simulink library "carnot"  (R2018b)
settings: Solver=VariableStepAuto  StartTime=0.0  StopTime=10.0  RelTol=1e-3
undefined symbols (not defined in the file or in its folder): A, A_earth, acol, Acol, ActPower1, ActPower2, ActPower3, Ad, Ad0, Ar, Au, Au0, Azimuth_Angle, B, Bd, Bd0, Br, Bu, Bu0, C, c1, c2, c3, c33, c4, c5, c6, CarnotCallbacks_Density, CarnotCallbacks_Enthalpy, CarnotCallbacks_Enthalpy2Temperature, CarnotCallbacks_Entropy, CarnotCallbacks_Evaporation_Enthalpy, CarnotCallbacks_GlobalMessageLevel, CarnotCallbacks_Grashof, CarnotCallbacks_Heat_Capacity, CarnotCallbacks_Kinematic_Viscosity, CarnotCallbacks_PMV_PPD, CarnotCallbacks_Prandtl, CarnotCallbacks_Saturation_Property, CarnotCallbacks_Saturation_Temperature, CarnotCallbacks_Saturation_Value_Water, CarnotCallbacks_Specific_Volume, CarnotCallbacks_Thermal_Conductivity, CarnotCallbacks_Vapour_Content, CarnotCallbacks_Vapour_Pressure, Cd, Cdl, Cr, Cu, Davies, Dd, DE_TRY2010_04_averageYear, delta_grd, density, DiameterLastPiece, dl, DPConstant, DPLinear, DPQuadratic, Dr ... (+59)
libraries: $bdroot x429, simulink x36, simulink_extras x12
(part 12 of 22)

== system carnot/Toolbox/Average ==
  input : Inport
  time : Inport  Port=2
  enable : Inport  Port=3
  Demux1 : Demux  Outputs=[-1 1 1]
  Mux : Mux  Inputs=3
  S-Function3 : S-Function  FunctionName=average  Parameters=delta_t offset_flag enable_flag  SFunctionDeploymentMode=off  EnableBusSupport=off  SFcnStateName=D_LAST_OUTPUT
      settings: SFcnIsStateOwnerBlock=on
  average : Outport
  output time : Outport  Port=2
  pulse : Outport  Port=3
  wires:
  Mux/1 -> S-Function3/1
  enable/1 -> Mux/3
  input/1 -> Mux/1
  S-Function3/1 -> Demux1/1
  Demux1/2 -> output time/1
  time/1 -> Mux/2
  Demux1/3 -> pulse/1
  Demux1/1 -> average/1

== system carnot/Toolbox/Economy_Ecology ==
  note: mass of fuel in kg
  note: thermal energy in J
  note: electric energy in J
  note: fuel costs
  note: mass of produced H2O
  note: mass of produced CO2
  note: mass of produced O2
  note: mass of produced SO2
  note: mass of produced N2
  note: mass of produced NOx
  note: mass of produced CO
  note: mass of produced CxHy
  eco : Inport
  Count_Working_Time : $bdroot/Toolbox/Count_Working_Time
  Demux1 : Demux  Outputs=12
  Display : Display
  Integrator : Integrator
  Mux : Mux  Inputs=12
  Mux1 : Mux  Inputs=2
  Selector : Selector  InputPortWidth=16  IndexOptions=Index vector (dialog)  Indices=[3 5:15]  OutputSizes=1
  Selector1 : Selector  InputPortWidth=12  IndexOptions=Index vector (dialog)  Indices=[1]  OutputSizes=1
  Terminator : Terminator
  Terminator1 : Terminator
  Terminator2 : Terminator
  To Workspace : ToWorkspace  VariableName=input_annual_costs  SampleTime=-1
      settings: MaxDataPoints=1
  wires:
  Count_Working_Time/3 -> Terminator2/1
  Count_Working_Time/2 -> Terminator1/1
  Count_Working_Time/1 -> Terminator/1
  Count_Working_Time/4 -> Mux1/2  "Run time"
  Demux1/4 -> Mux1/1, Mux/4  "costs"
  Demux1/1 -> Mux/1  "m_fuel"
  Selector1/1 -> Count_Working_Time/1
  Selector/1 -> Selector1/1, Integrator/1
  Mux1/1 -> To Workspace/1
  Mux/1 -> Display/1
  Demux1/3 -> Mux/3  "E_electric"
  Demux1/2 -> Mux/2  "Qtherm"
  Demux1/10 -> Mux/10  "NOx"
  Demux1/11 -> Mux/11  "CO"
  Demux1/12 -> Mux/12  "CxHy"
  Demux1/9 -> Mux/9  "N2"
  Demux1/6 -> Mux/6  "CO2"
  Integrator/1 -> Demux1/1
  eco/1 -> Selector/1
  Demux1/7 -> Mux/7  "O2"
  Demux1/5 -> Mux/5  "H20"
  Demux1/8 -> Mux/8  "SO2"

== system carnot/Toolbox/GlobalMessageLevel ==

== system carnot/Toolbox/ModelDoc ==

== system carnot/Toolbox/RealDate ==
  S-Function3 : S-Function  FunctionName=systemdate  Parameters=form  SFunctionDeploymentMode=off  EnableBusSupport=off
  date : Outport
  wires:
  S-Function3/1 -> date/1

== system carnot/Toolbox/RealTime ==
  S-Function3 : S-Function  FunctionName=systemtime  SFunctionDeploymentMode=off  EnableBusSupport=off
  time : Outport
  wires:
  S-Function3/1 -> time/1

== system carnot/Toolbox/RealTimePulse ==
  In : Inport
  S-Function : S-Function  FunctionName=monoflop_realtime  Parameters=time typ  SFunctionDeploymentMode=off  EnableBusSupport=off
  Out : Outport
  wires:
  In/1 -> S-Function/1
  S-Function/1 -> Out/1

== system carnot/Toolbox/SystemPulse ==
  enable pulse : Inport
  Mux : Mux  Inputs=2
  S-Function3 : S-Function  FunctionName=systempulse  Parameters=datecheck enable_flag  SFunctionDeploymentMode=off  EnableBusSupport=off
  position6 : Constant  Value=[date period pulsewidth]
  pulse : Outport
  wires:
  Mux/1 -> S-Function3/1
  enable pulse/1 -> Mux/2
  S-Function3/1 -> pulse/1
  position6/1 -> Mux/1

== system carnot/Toolbox/THB2THV ==
  THB : Inport  OutDataTypeStr=Bus: THB
  Bus Selector : BusSelector  OutputSignals=ID,Temperature,MassFlow,Pressure,FluidType,FluidMix,DiameterLastPiece,DPConstant,DPLinear,DPQuadratic,HydraulicInductance,GeodeticHeight,FluidMix2,FluidMix3
  Ground : Ground
  Mux : Mux  Inputs=[1 1 1 1 1 1 1 1 1 1 1 1 1 1 6]
  THV : Outport
  wires:
  Bus Selector/14 -> Mux/14  "<FluidMix3>"
  Bus Selector/13 -> Mux/13  "<FluidMix2>"
  THB/1 -> Bus Selector/1
  Mux/1 -> THV/1
  Bus Selector/1 -> Mux/1  "<ID>"
  Bus Selector/2 -> Mux/2  "<Temperature>"
  Bus Selector/3 -> Mux/3  "<MassFlow>"
  Bus Selector/4 -> Mux/4  "<Pressure>"
  Bus Selector/5 -> Mux/5  "<FluidType>"
  Bus Selector/6 -> Mux/6  "<FluidMix>"
  Bus Selector/7 -> Mux/7  "<DiameterLastPiece>"
  Bus Selector/8 -> Mux/8  "<DPConstant>"
  Bus Selector/9 -> Mux/9  "<DPLinear>"
  Bus Selector/10 -> Mux/10  "<DPQuadratic>"
  Bus Selector/11 -> Mux/11  "<HydraulicInductance>"
  Bus Selector/12 -> Mux/12  "<GeodeticHeight>"
  Ground/1 -> Mux/15

== system carnot/Toolbox/THBMemory ==
  THB_in : Inport  OutDataTypeStr=Bus: THB
  Bus Creator : BusCreator  Inputs=12
  Bus Selector6 : BusSelector  OutputSignals=ID,Temperature,MassFlow,Pressure,FluidType,FluidMix,DiameterLastPiece,DPConstant,DPLinear,DPQuadratic,HydraulicInductance,GeodeticHeight
  Memory_DPConstant : Memory  InitialCondition=c
  Memory_DPLinear : Memory  InitialCondition=l
  Memory_DPQuadratic : Memory  InitialCondition=q
  Memory_DiameterLastPiece : Memory  InitialCondition=d
  Memory_FluidMix : Memory  InitialCondition=FluidMix
  Memory_FluidType : Memory  InitialCondition=FluidType
  Memory_GeodeticHeight : Memory  InitialCondition=H
  Memory_HydraulicInductance : Memory  InitialCondition=LH
  Memory_ID : Memory  InitialCondition=ID
  Memory_MassFlow : Memory  InitialCondition=mdot
  Memory_Pressure : Memory  InitialCondition=p
  Memory_Temperature : Memory  InitialCondition=T
  THB_out : Outport
  wires:
  Bus Selector6/12 -> Memory_GeodeticHeight/1  "<GeodeticHeight>"
  Memory_GeodeticHeight/1 -> Bus Creator/12  "GeodeticHeight"
  Bus Selector6/1 -> Memory_ID/1  "<ID>"
  Memory_ID/1 -> Bus Creator/1  "ID"
  Bus Selector6/2 -> Memory_Temperature/1  "<Temperature>"
  Memory_Temperature/1 -> Bus Creator/2  "Temperature"
  Bus Selector6/3 -> Memory_MassFlow/1  "<MassFlow>"
  Memory_MassFlow/1 -> Bus Creator/3  "MassFlow"
  Bus Selector6/4 -> Memory_Pressure/1  "<Pressure>"
  Memory_Pressure/1 -> Bus Creator/4  "Pressure"
  Bus Selector6/5 -> Memory_FluidType/1  "<FluidType>"
  Memory_FluidType/1 -> Bus Creator/5  "FluidType"
  Bus Selector6/6 -> Memory_FluidMix/1  "<FluidMix>"
  Memory_FluidMix/1 -> Bus Creator/6  "FluidMix"
  Bus Selector6/7 -> Memory_DiameterLastPiece/1  "<DiameterLastPiece>"
  Memory_DiameterLastPiece/1 -> Bus Creator/7  "DiameterLastPiece"
  Bus Selector6/8 -> Memory_DPConstant/1  "<DPConstant>"
  Memory_DPConstant/1 -> Bus Creator/8  "DPConstant"
  Bus Selector6/9 -> Memory_DPLinear/1  "<DPLinear>"
  Memory_DPLinear/1 -> Bus Creator/9  "DPLinear"
  Bus Selector6/10 -> Memory_DPQuadratic/1  "<DPQuadratic>"
  Memory_DPQuadratic/1 -> Bus Creator/10  "DPQuadratic"
  Bus Selector6/11 -> Memory_HydraulicInductance/1  "<HydraulicInductance>"
  Memory_HydraulicInductance/1 -> Bus Creator/11  "HydraulicInductance"
  Bus Creator/1 -> THB_out/1
  THB_in/1 -> Bus Selector6/1

== system carnot/Toolbox/THV2THB ==
  THV : Inport
  Bus Creator : BusCreator  Inputs=14  OutDataTypeStr=Bus: THB
  Demux : Demux  Outputs=[1 1 1 1 1 1 1 1 1 1 1 1 1 1 6]
  Terminator : Terminator
  THB : Outport
  wires:
  [FluidMix3] -> Bus Creator/8  "FluidMix3"
  [FluidMix2] -> Bus Creator/7  "FluidMix2"
  Demux/14 -> [FluidMix3]  "FluidMix3"
  Demux/13 -> [FluidMix2]  "FluidMix2"
  Demux/15 -> Terminator/1
  Demux/12 -> Bus Creator/14  "GeodeticHeight"
  Demux/10 -> Bus Creator/12  "DPQuadratic"
  Demux/9 -> Bus Creator/11  "DPLinear"
  Demux/8 -> Bus Creator/10  "DPConstant"
  Demux/7 -> Bus Creator/9  "DiameterLastPiece"
  Demux/6 -> Bus Creator/6  "FluidMix"
  Demux/5 -> Bus Creator/5  "FluidType"
  Bus Creator/1 -> THB/1
  Demux/4 -> Bus Creator/4  "Pressure"
  Demux/3 -> Bus Creator/3  "MassFlow"
  Demux/1 -> Bus Creator/1  "ID"
  Demux/2 -> Bus Creator/2  "Temperature"
  THV/1 -> Demux/1
  Demux/11 -> Bus Creator/13  "HydraulicInductance"

== system carnot/Toolbox/UnitConv ==
  In : Inport
  S-Function : S-Function  FunctionName=unitconv_s  Parameters=input_unit output_unit  SFunctionDeploymentMode=off  EnableBusSupport=off
  Out : Outport
  wires:
  In/1 -> S-Function/1
  S-Function/1 -> Out/1

== system carnot/Toolbox/UnitConv_Temperature ==
  Tinit : Inport
  S-Function : S-Function  FunctionName=unitconv_temperature_s  Parameters=ini_unit, fin_unit  SFunctionDeploymentMode=off  EnableBusSupport=off
  Tfinal : Outport
  wires:
  S-Function/1 -> Tfinal/1
  Tinit/1 -> S-Function/1

== system carnot/Toolbox/WDB2Weather ==
  WDB : Inport
  Bus Selector1 : BusSelector  OutputSignals=TimeValueComment,Zenith_Angle,Azimuth_Angle,Solar_Radiation_beam_normal,Solar_Radiation_diffuse_horizontal,Temperature_Ambient,Temperature_Sky_Radiation,Relative_Humidity,Precipitation,Cloud_Index,Station_Pressure,Wind_Speed,Wind_Direction,Incidence_Angle_sun,Incidence_Angle_longitudinal,Incidence_Angle_transversal,Solar_Radiation_direct_surface,Solar_Radiation_diffuse_surface
  Mux : Mux  Inputs=18
  weather : Outport
  wires:
  Bus Selector1/1 -> Mux/1  "<TimeValueComment>"
  Bus Selector1/2 -> Mux/2  "<Zenith_Angle>"
  Bus Selector1/3 -> Mux/3  "<Azimuth_Angle>"
  Bus Selector1/4 -> Mux/4  "<Solar_Radiation_beam_normal>"
  Bus Selector1/5 -> Mux/5  "<Solar_Radiation_diffuse_horizontal>"
  Bus Selector1/6 -> Mux/6  "<Temperature_Ambient>"
  Bus Selector1/7 -> Mux/7  "<Temperature_Sky_Radiation>"
  Bus Selector1/8 -> Mux/8  "<Relative_Humidity>"
  Bus Selector1/9 -> Mux/9  "<Precipitation>"
  Bus Selector1/10 -> Mux/10  "<Cloud_Index>"
  Bus Selector1/11 -> Mux/11  "<Station_Pressure>"
  Bus Selector1/12 -> Mux/12  "<Wind_Speed>"
  Bus Selector1/13 -> Mux/13  "<Wind_Direction>"
  Bus Selector1/14 -> Mux/14  "<Incidence_Angle_sun>"
  Bus Selector1/15 -> Mux/15  "<Incidence_Angle_longitudinal>"
  Bus Selector1/16 -> Mux/16  "<Incidence_Angle_transversal>"
  Bus Selector1/17 -> Mux/17  "<Solar_Radiation_direct_surface>"
  Bus Selector1/18 -> Mux/18  "<Solar_Radiation_diffuse_surface>"
  WDB/1 -> Bus Selector1/1
  Mux/1 -> weather/1

== system carnot/Toolbox/Wait ==
  S-Function3 : S-Function  FunctionName=wait  Parameters=date(1) date(2) date(3) date(4) date(5) wtime  SFunctionDeploymentMode=off  EnableBusSupport=off

== system carnot/Toolbox/Weather2WDB ==
  weather : Inport
  Demux : Demux  Outputs=18
  WDB_Creator : $bdroot/Basic/Weather_and_Sun/WDB_Creator
  WDB : Outport
  wires:
  weather/1 -> Demux/1
  WDB_Creator/1 -> WDB/1
  Demux/1 -> WDB_Creator/1  "time_value"
  Demux/2 -> WDB_Creator/2  "zenith"
  Demux/3 -> WDB_Creator/3  "azimuth"
  Demux/4 -> WDB_Creator/4  "I_beam_normal"
  Demux/5 -> WDB_Creator/5  "I_diffuse_horizontal"
  Demux/6 -> WDB_Creator/6  "Tamb"
  Demux/7 -> WDB_Creator/7  "Tsky"
  Demux/8 -> WDB_Creator/8  "relative_humidity"
  Demux/9 -> WDB_Creator/9  "precipitation"
  Demux/10 -> WDB_Creator/10  "cloud_index"
  Demux/11 -> WDB_Creator/11  "pressure"
  Demux/12 -> WDB_Creator/12  "wind_speed"
  Demux/13 -> WDB_Creator/13  "wind_direction"
  Demux/14 -> WDB_Creator/14  "incidence_angle"
  Demux/15 -> WDB_Creator/15  "longitudinal_angle"
  Demux/16 -> WDB_Creator/16  "transversal_angle"
  Demux/17 -> WDB_Creator/17  "I_direct_surface"
  Demux/18 -> WDB_Creator/18  "I_diffuse_surface"

== system carnot/Toolbox/write_txt_file ==
  In : Inport
  enable : Inport  Port=2
  Mux1 : Mux  Inputs=2
  S-Function : S-Function  FunctionName=write_txt_file  Parameters=clear filename  SFunctionDeploymentMode=off  EnableBusSupport=off
  Terminator : Terminator
  wires:
  enable/1 -> Mux1/2
  In/1 -> Mux1/1
  Mux1/1 -> S-Function/1
  S-Function/1 -> Terminator/1

== system carnot/Weather/Add_Solar_Position ==
  WDB_in : Inport
  Bus Assignment : BusAssignment  AssignedSignals=Zenith_Angle,Azimuth_Angle
  Demux : Demux  Outputs=2
  Solar_Position : $bdroot/Basic/Weather_and_Sun/Solar_Position  lati=lati  longi=longi  timezone=timezone
  WDB : Outport
  wires:
  Bus Assignment/1 -> WDB/1
  Demux/2 -> Bus Assignment/3
  Demux/1 -> Bus Assignment/2
  WDB_in/1 -> Bus Assignment/1
  Solar_Position/1 -> Demux/1  "zenith, azimuth"

== system carnot/Weather/DWD_TRY_Radiation_Filter ==
  WDB : Inport
  Bus Assignment : BusAssignment  AssignedSignals=Solar_Radiation_beam_normal,Solar_Radiation_diffuse_horizontal,Solar_Radiation_direct_surface,Solar_Radiation_diffuse_surface
  Bus Selector1 : BusSelector  OutputSignals=Incidence_Angle_sun
  Bus Selector2 : BusSelector  OutputSignals=Solar_Radiation_beam_normal,Solar_Radiation_diffuse_horizontal,Solar_Radiation_direct_surface,Solar_Radiation_diffuse_surface
  Degrees to Radians : simulink_extras/Transformations/Degrees to Radians
  Demux : Demux  Outputs=3
  Gain : Gain  Gain=f
  MinMax : MinMax  Inputs=2
  Mux : Mux  Inputs=3
  Product : Product
  Saturation : Saturate  UpperLimit=inf  LowerLimit=0
  Trigonometric Function : Trigonometry  Operator=cos
  WDB_filter : Outport
  wires:
  Saturation/1 -> MinMax/2
  Gain/1 -> Product/2
  Product/1 -> Saturation/1
  Trigonometric Function/1 -> Gain/1
  Degrees to Radians/1 -> Trigonometric Function/1
  Bus Selector2/1 -> MinMax/1, Product/1  "<Solar_Radiation_beam_normal>"
  Bus Selector2/2 -> Mux/1  "<Solar_Radiation_diffuse_horizontal>"
  MinMax/1 -> Bus Assignment/2  "Solar_Radiation_beam_normal"
  Demux/1 -> Bus Assignment/3  "Solar_Radiation_diffuse_horizontal"
  Demux/3 -> Bus Assignment/5  "Solar_Radiation_diffuse_surface"
  Demux/2 -> Bus Assignment/4  "Solar_Radiation_direct_surface"
  Bus Selector2/4 -> Mux/3  "<Solar_Radiation_diffuse_surface>"
  Bus Selector2/3 -> Mux/2  "<Solar_Radiation_direct_surface>"
  Mux/1 -> Demux/1
  Bus Selector1/1 -> Degrees to Radians/1  "<Incidence_Angle_sun>"
  Bus Assignment/1 -> WDB_filter/1
  WDB/1 -> Bus Assignment/1, Bus Selector1/1, Bus Selector2/1

== system carnot/Weather/Fixed_Surface ==
  Bus Creator : BusCreator  Inputs=3
  collector position : Constant  Value=colangle
  collector position1 : Constant  Value=colazi
  collector position2 : Constant  Value=colrot
  position : Outport
  wires:
  collector position2/1 -> Bus Creator/3  "rotation"
  collector position1/1 -> Bus Creator/2  "azimut"
  collector position/1 -> Bus Creator/1  "inclination"
  Bus Creator/1 -> position/1

== system carnot/Weather/Radiation_on_Inclined_Surface ==
  WDB_in : Inport
  position : Inport  Port=2
  WDB2Weather : $bdroot/Toolbox/WDB2Weather
  WDB_Creator : $bdroot/Basic/Weather_and_Sun/WDB_Creator
  radiation_on_surface : S-Function  FunctionName=surfrad  Parameters=sky,reflect  SFunctionDeploymentMode=off  EnableBusSupport=off
  WDB_out : Outport
  wires:
  WDB2Weather/1 -> radiation_on_surface/1
  WDB_Creator/1 -> WDB_out/1
  radiation_on_surface/18 -> WDB_Creator/18  "Solar_Radiation_diffuse_surface"
  radiation_on_surface/17 -> WDB_Creator/17  "Solar_Radiation_direct_surface"
  radiation_on_surface/16 -> WDB_Creator/16  "Incidence_Angle_transversal"
  radiation_on_surface/15 -> WDB_Creator/15  "Incidence_Angle_longitudinal"
  radiation_on_surface/14 -> WDB_Creator/14  "Incidence_Angle_sun"
  radiation_on_surface/13 -> WDB_Creator/13  "Wind_Direction"
  radiation_on_surface/12 -> WDB_Creator/12  "Wind_Speed"
  radiation_on_surface/11 -> WDB_Creator/11  "Station_Pressure"
  radiation_on_surface/10 -> WDB_Creator/10  "Cloud_Index"
  radiation_on_surface/9 -> WDB_Creator/9  "Precipitation"
  radiation_on_surface/8 -> WDB_Creator/8  "Relative_Humidity"
  radiation_on_surface/7 -> WDB_Creator/7  "Temperature_Sky_Radiation"
  radiation_on_surface/6 -> WDB_Creator/6  "Temperature_Ambient"
  radiation_on_surface/5 -> WDB_Creator/5  "Solar_Radiation_diffuse_horizontal"
  radiation_on_surface/4 -> WDB_Creator/4  "Solar_Radiation_beam_normal"
  radiation_on_surface/3 -> WDB_Creator/3  "Azimuth_Angle"
  radiation_on_surface/2 -> WDB_Creator/2  "Zenith_Angle"
  radiation_on_surface/1 -> WDB_Creator/1  "TimeValueComment"
  WDB_in/1 -> WDB2Weather/1
  position/1 -> radiation_on_surface/2

== system carnot/Weather/Select_Weather ==
  weather : Inport
  Selector : Selector  InputPortWidth=18  IndexOptions=Index vector (dialog)  Indices=v  OutputSizes=1
  data : Outport  InitialOutput=0
  wires:
  Selector/1 -> data/1
  weather/1 -> Selector/1

== system carnot/Weather/Tracked_Surface ==
  WDB : Inport
  Bus Creator : BusCreator  Inputs=3
  Bus Selector : BusSelector  OutputSignals=Zenith_Angle,Azimuth_Angle
  Demux : Demux  Outputs=3
  Mux : Mux  Inputs=2
  s-function : S-Function  FunctionName=tracking  Parameters=tracktype time inc azi rot  SFunctionDeploymentMode=off  EnableBusSupport=off
  position : Outport
  wires:
  Bus Selector/2 -> Mux/2  "<Azimuth_Angle>"
  Bus Selector/1 -> Mux/1  "<Zenith_Angle>"
  Mux/1 -> s-function/1
  WDB/1 -> Bus Selector/1
  Demux/1 -> Bus Creator/1  "inclination"
  Demux/2 -> Bus Creator/2  "azimut"
  Demux/3 -> Bus Creator/3  "rotation"
  s-function/1 -> Demux/1
  Bus Creator/1 -> position/1

== system carnot/Weather/WDB2THB ==
  WDB : Inport
  Bus Assignment : BusAssignment  AssignedSignals=Temperature,Pressure,FluidMix
  Bus Selector : BusSelector  OutputSignals=Temperature_Ambient,Relative_Humidity,Station_Pressure
  Constant_THB : $bdroot/Source/Simple/Constant_THB  t=10  mdot=0  p=1e5  mID=No Pressure Drop  fluid=Air  mix=0  mix2=0  mix3=0  dia=dia  hgt=0
  RelHum2x : $bdroot/Basic/Material_Properties/RelHum2x
  THB : Outport
  wires:
  RelHum2x/1 -> Bus Assignment/4
  Bus Selector/3 -> Bus Assignment/3, RelHum2x/2  "<Station_Pressure>"
  Bus Selector/2 -> RelHum2x/3  "<Relative_Humidity>"
  Bus Selector/1 -> Bus Assignment/2, RelHum2x/1  "<Temperature_Ambient>"
  Bus Assignment/1 -> THB/1
  Constant_THB/1 -> Bus Assignment/1
  WDB/1 -> Bus Selector/1

== system carnot/Weather/Weather_Datafile ==
  Constant : Constant
  FromWorkspace : FromWorkspace  VariableName=VariableName  SampleTime=0  OutputAfterFinalValue=Holding final value
  Terminator : Terminator
  UnitDelay : UnitDelay  SampleTime=SampleTime
  Weather2WDB : $bdroot/Toolbox/Weather2WDB
  WDB : Outport
  wires:
  Weather2WDB/1 -> WDB/1  "WDB"
  FromWorkspace/1 -> Weather2WDB/1
  Constant/1 -> UnitDelay/1
  UnitDelay/1 -> Terminator/1

== system carnot/Weather/Weather_Simple_Model ==
  Bias : Bias  Bias=deltaTsky
  Compare To Constant : simulink/Logic and Bit Operations/Compare To Constant  relop=<  const=90  OutDataTypeStr=uint8
  Constant : Constant
  Data Type Conversion : DataTypeConversion
  Demux : Demux  Outputs=2
  Fixed_Surface : $bdroot/Weather/Fixed_Surface  colangle=colangle  colazi=colazi  colrot=colrot
  Gain : Gain  Gain=Ibn
  Gain1 : Gain  Gain=Idg
  Idiffuse_surface : Constant  Value=-9999
  Idirect_surface : Constant  Value=-9999
  Radiation_on_Inclined_Surface : $bdroot/Weather/Radiation_on_Inclined_Surface  sky=Perez 1990  reflect=0.2
  Solar_Position : $bdroot/Basic/Weather_and_Sun/Solar_Position  lati=lat  longi=longi  timezone=timezone
  Tamb : Constant  Value=tamb
  Terminator : Terminator
  Unit Delay : UnitDelay  SampleTime=3600
  WDB_Creator : $bdroot/Basic/Weather_and_Sun/WDB_Creator
  cloud [0..1] : Constant  Value=cloud
  comment : Constant  Value=-9999
  "direction [0 = north, 90 = east]" : Constant  Value=wdir
  incidence : Constant  Value=-9999
  precip [m/s] : Constant  Value=precip
  pressure [Pa] : Constant  Value=p
  relative_humidity in % : Constant  Value=rh
  tetap : Constant  Value=-9999
  tetas : Constant  Value=-9999
  windspeed [m/s] : Constant  Value=vw
  WDB : Outport
  wires:
  WDB_Creator/1 -> Radiation_on_Inclined_Surface/1
  Radiation_on_Inclined_Surface/1 -> WDB/1
  Fixed_Surface/1 -> Radiation_on_Inclined_Surface/2
  Gain/1 -> WDB_Creator/4  "Solar_Radiation_beam_normal"
  Solar_Position/1 -> Demux/1
  comment/1 -> WDB_Creator/1  "TimeValueComment"
  Demux/1 -> WDB_Creator/2, Compare To Constant/1  "Zenith_Angle"
  Demux/2 -> WDB_Creator/3  "Azimuth_Angle"
  Compare To Constant/1 -> Data Type Conversion/1
  Gain1/1 -> WDB_Creator/5  "Solar_Radiation_diffuse_horizontal"
  Tamb/1 -> WDB_Creator/6, Bias/1  "Temperature_Ambient"
  Bias/1 -> WDB_Creator/7  "Temparature_Sky_Radiation"
  relative_humidity in %/1 -> WDB_Creator/8  "Relative_Humidity"
  precip [m/s]/1 -> WDB_Creator/9  "Precipitation"
  cloud [0..1]/1 -> WDB_Creator/10  "Cloud_Index"
  pressure [Pa]/1 -> WDB_Creator/11  "Station_Pressure"
  windspeed [m/s]/1 -> WDB_Creator/12  "Wind_Speed"
  "direction [0 = north, 90 = east]"/1 -> WDB_Creator/13  "Wind_Direction"
  incidence/1 -> WDB_Creator/14  "Incidence_Angle_sun"
  tetap/1 -> WDB_Creator/15  "Incidence_Angle_longitudinal"
  tetas/1 -> WDB_Creator/16  "Incidence_Angle_transversal"
  Idirect_surface/1 -> WDB_Creator/17  "Solar_Radiation_direct_surface"
  Idiffuse_surface/1 -> WDB_Creator/18  "Solar_Radiation_diffuse_surface"
  Data Type Conversion/1 -> Gain1/1, Gain/1
  Constant/1 -> Unit Delay/1
  Unit Delay/1 -> Terminator/1

== system carnot/Weather/Weather_from_Workspace ==
  Constant : Constant
  From_Workspace : FromWorkspace  VariableName=DE_TRY2010_06_averageYear  SampleTime=0  OutputAfterFinalValue=Setting to zero
  Terminator : Terminator
  Unit Delay : UnitDelay  SampleTime=t_sample
  Weather2WDB : $bdroot/Toolbox/Weather2WDB
  WDB : Outport
  wires:
  From_Workspace/1 -> Weather2WDB/1
  Constant/1 -> Unit Delay/1
  Unit Delay/1 -> Terminator/1
  Weather2WDB/1 -> WDB/1

== system carnot/Basic/Electric/EBCreator ==
  ID : Inport
  Frequency : Inport  Port=2
  Voltage1 : Inport  Port=3
  ActPower1 : Inport  Port=4
  PowerFactor1 : Inport  Port=5
  Voltage2 : Inport  Port=6
  ActPower2 : Inport  Port=7
  PowerFactor2 : Inport  Port=8
  Voltage3 : Inport  Port=9
  ActPower3 : Inport  Port=10
  PowerFactor3 : Inport  Port=11
  BusCreator : BusCreator  Inputs=11  OutDataTypeStr=Bus: EB
      settings: InheritFromInputs=off
  EB : Outport  OutDataTypeStr=Bus: EB
  wires:
  PowerFactor3/1 -> BusCreator/11  "PowerFactor3"
  ActPower3/1 -> BusCreator/10  "ActPower3"
  Voltage3/1 -> BusCreator/9  "Voltage3"
  PowerFactor2/1 -> BusCreator/8  "PowerFactor2"
  ActPower2/1 -> BusCreator/7  "ActPower2"
  Voltage2/1 -> BusCreator/6  "Voltage2"
  PowerFactor1/1 -> BusCreator/5  "PowerFactor1"
  ActPower1/1 -> BusCreator/4  "ActPower1"
  Voltage1/1 -> BusCreator/3  "Voltage1"
  Frequency/1 -> BusCreator/2  "Frequency"
  ID/1 -> BusCreator/1  "ID"
  BusCreator/1 -> EB/1

== system carnot/Basic/Electric/basic_EB ==
  Bus Creator : BusCreator  InitFcn=load THB.mat  Inputs=11  OutDataTypeStr=Bus: EB
      settings: InheritFromInputs=off
  ID : Constant  Value=ID  mask{eID=Power only}
      mask prompts: eID "ID for electric calculation"
      mask init:
      | ID = eID;
      mask TypeOptions eID: Power only | DC | AC_1P | AC_3P
  f : Constant  Value=f
  p1 : Constant  Value=p1
  p2 : Constant  Value=p2
  p3 : Constant  Value=p3
  pf1 : Constant  Value=pf1
  pf2 : Constant  Value=pf2
  pf3 : Constant  Value=pf3
  v1 : Constant  Value=v1
  v2 : Constant  Value=v2
  v3 : Constant  Value=v3
  EB : Outport
  wires:
  pf2/1 -> Bus Creator/8  "PowerFactor2"
  p2/1 -> Bus Creator/7  "ActPower2"
  pf3/1 -> Bus Creator/11  "PowerFactor3"
  v3/1 -> Bus Creator/9  "Voltage3"
  p3/1 -> Bus Creator/10  "ActPower3"
  Bus Creator/1 -> EB/1
  ID/1 -> Bus Creator/1  "ID"
  v1/1 -> Bus Creator/3  "Voltage1"
  p1/1 -> Bus Creator/4  "ActPower1"
  pf1/1 -> Bus Creator/5  "PowerFactor1"
  f/1 -> Bus Creator/2  "Freq"
  v2/1 -> Bus Creator/6  "Voltage2"

== system carnot/Basic/Electric/basic_create_EB ==
  voltage : Inport
  active power : Inport  Port=2
  EB_set_power : $bdroot/Source/Simple/EB_set_power
  EB_set_voltage : $bdroot/Source/Simple/EB_set_voltage
  basic_EB : $bdroot/Basic/Electric/basic_EB  eID=Power only  f=f  v1=230  p1=0  pf1=pf1  v2=230  p2=0  pf2=pf2  v3=230  p3=0  pf3=pf3
  EB : Outport
  wires:
  EB_set_power/1 -> EB/1
  voltage/1 -> EB_set_voltage/2
  active power/1 -> EB_set_power/2
  basic_EB/1 -> EB_set_voltage/1
  EB_set_voltage/1 -> EB_set_power/1

== system carnot/Basic/Heat_Transfer/HeatTransfer2Ground_ISO13370 ==
  note: heat transfer
      | to ground
  note: effectie thermal resistance
      | of the ground
  note: ISO 13370:2007 "Slab on Ground"
  Afloor : Constant  Value=slablength*slabwidth
  Bfloor : Constant  Value=(slablength*slabwidth)/(slablength+slabwidth)
  COS_Texternal : Fcn  Expr=cos(2*pi*((u(2)-tshift)/3600-u(1))/8760)
  COS_Tinternal : Fcn  Expr=cos(2*pi*((u(2)-tshift)/3600-u(1))/8760)
  Clock : Clock
  Clock2 : Clock
  Lpe*deltathetae : Fcn  Expr=deltathetae*(0.37*u(1)*cond_ground*log(u(2)/u(3)+1))
  Lpi*deltathetai : Fcn  Expr=deltathetai*(u(3)*cond_ground/u(1)*sqrt(2/((1+u(2)/u(1))^2+1)))
  Ls*(thetae-thetai) : Fcn  Expr=(u(1)*u(3)+u(2)*gammat)*(Tmeanoutside-Tmeaninside)
  Mux2 : Mux  Inputs=2
  Mux3 : Mux  Inputs=3
  Mux4 : Mux  Inputs=3
  Mux5 : Mux  Inputs=2
  Mux6 : Mux  Inputs=2
  Mux7 : Mux  Inputs=3
  Perimeter : Constant  Value=2*(slablength+slabwidth)
  Product1 : Product  SaturateOnIntegerOverflow=on  RndMeth=Zero  InputSameDT=on  OutDataTypeStr=Inherit: Same as first input
  Product3 : Product  SaturateOnIntegerOverflow=on  RndMeth=Zero  InputSameDT=on  OutDataTypeStr=Inherit: Same as first input
  Rground : Fcn  Expr=0.457*u/cond_ground
  Sum6 : Sum  Inputs=--+
  Usteady : Fcn  Expr=1/(1/utot+dwall/cond_ground+u)
  alpha : Fcn  Expr=(1.5-12/(2*pi)*atan(u(1)/(u(1)+u(2))))*8760/12
  beta : Fcn  Expr=(1.5-0.42*log(u(2)/u(1)+1))*8760/12
  delta_grd : Constant  Value=sqrt((8760*3600*cond_ground)/(pi*rho_ground*cp_ground))
  dt : Constant  Value=dwall+cond_ground/utot
  Qdot : Outport
  wires:
  Rground/1 -> Usteady/1
  Bfloor/1 -> Rground/1
  dt/1 -> Mux7/3, Mux4/1, Mux2/1
  delta_grd/1 -> Mux2/2, Mux4/2, Mux7/2
  Mux2/1 -> alpha/1, beta/1
  Mux3/1 -> Ls*(thetae-thetai)/1
  Afloor/1 -> Mux4/3, Mux3/1  "m2"
  Perimeter/1 -> Mux3/2, Mux7/1
  Usteady/1 -> Mux3/3
  Mux4/1 -> Lpi*deltathetai/1
  Lpi*deltathetai/1 -> Product3/2
  alpha/1 -> Mux5/1  "h"
  Clock/1 -> Mux5/2  "s"
  Mux5/1 -> COS_Tinternal/1
  COS_Tinternal/1 -> Product3/1
  Product3/1 -> Sum6/2
  Ls*(thetae-thetai)/1 -> Sum6/3
  beta/1 -> Mux6/1  "h"
  Clock2/1 -> Mux6/2  "s"
  Mux6/1 -> COS_Texternal/1
  COS_Texternal/1 -> Product1/1
  Lpe*deltathetae/1 -> Product1/2
  Product1/1 -> Sum6/1
  Mux7/1 -> Lpe*deltathetae/1
  Sum6/1 -> Qdot/1  "W"

== system carnot/Basic/Heat_Transfer/HeatTransfer2Ground_Simple ==
  Troom : Inport
  Sum2 : Sum  Inputs=+-  SaturateOnIntegerOverflow=on  InputSameDT=on  OutDataTypeStr=Inherit: Same as first input
  UAground : Gain  Gain=UAground  SaturateOnIntegerOverflow=on  OutDataTypeStr=Inherit: Same as input  ParamDataTypeStr=Inherit: Same as input
  const1 : Constant  Value=Tground
  Qdot : Outport
  wires:
  Sum2/1 -> UAground/1
  const1/1 -> Sum2/1
  UAground/1 -> Qdot/1
  Troom/1 -> Sum2/2

== system carnot/Basic/Heat_Transfer/alfa_ceiling ==
  note: (°C)
  note: (W/m^2)
  note: Convective and radiative heat transfer at the SURFACE OF A HORIZONTAL CEILING
  note: s: surface
      | c: convective
      | r: radiative
  note: CONVENTION:
      | Qdot > 0 and qdots < 0, if Ts > T (heat flows from wall surface to room node),
      | Qdot < 0 and qdots > 0, if Ts < T (heat flows from room node to wall surface).
  note: dynamic, convective heat transfer coefficients according to: Glück B.: Wärmeübergangskoeffizienten an thermisch aktiven Bauteiloberflächen
      | und der Übergang zu Basiskennlinien für die Wärmestromdichte; gi Gesundheits-Ingenieur; 128. Jahrgang 2007, Heft 1, Seiten 1-10
  Ts : Inport
  "[AIV]c" : Inport  Port=2
  1-D Lookup Table : Lookup_n-D  NumberOfTableDimensions=1  BreakpointsForDimension1=[-10 -0.01 0.01 10]  BeginIndexSearchUsingPreviousIndexResult=on  Table=[2 2 0.54 0.54]  InternalRulePriority=Speed  RndMeth=Simplest  InputSameDT=on
  Abs : Abs
  Constant : Constant  Value=0.31
  Demux : Demux  Outputs=[1 1 1 6]
  Ground : Ground
  Ground1 : Ground
  Ground2 : Ground
  Math Function : Math  Operator=pow  SaturateOnIntegerOverflow=on
  Mux : Mux  Inputs=[1 1]
  Mux1 : Mux  Inputs=[4 1 1 2 5]
  Product1 : Product  Inputs=3  SaturateOnIntegerOverflow=on  RndMeth=Zero  InputSameDT=on  OutDataTypeStr=Inherit: Same as first input
  Sum : Sum  Inputs=-+  SaturateOnIntegerOverflow=on  InputSameDT=on  OutDataTypeStr=Inherit: Same as first input
  Sum1 : Sum  Inputs=+-  SaturateOnIntegerOverflow=on  InputSameDT=on  OutDataTypeStr=Inherit: Same as first input
  Sum2 : Sum  Inputs=--  SaturateOnIntegerOverflow=on  InputSameDT=on  OutDataTypeStr=Inherit: Same as first input
  Sum3 : Sum  Inputs=1  SaturateOnIntegerOverflow=on  InputSameDT=on  OutDataTypeStr=Inherit: Same as first input
  Terminator : Terminator
  Terminator1 : Terminator
  Urad*emissivity : Gain  Gain=5.6*emission_c  SaturateOnIntegerOverflow=on  OutDataTypeStr=Inherit: Same as input  ParamDataTypeStr=Inherit: Same as input
  active layers : Gain  Gain=active  SaturateOnIntegerOverflow=on  OutDataTypeStr=Inherit: Same as input  ParamDataTypeStr=Inherit: Same as input
  wallsurface : Gain  Gain=wallsurface  SaturateOnIntegerOverflow=on  OutDataTypeStr=Inherit: Same as input  ParamDataTypeStr=Inherit: Same as input
  qdots : Outport
  "[S]c" : Outport  Port=2
  wires:
  Math Function/1 -> Product1/3
  1-D Lookup Table/1 -> Product1/2  "coeff_upwards_downwards"
  Abs/1 -> Math Function/1
  Constant/1 -> Math Function/2
  active layers/1 -> Mux1/2
  Ground2/1 -> Mux1/3
  Mux1/1 -> "[S]c"/1
  Ground1/1 -> Mux1/5
  Ground/1 -> Mux1/1
  Sum3/1 -> active layers/1
  wallsurface/1 -> Sum3/1, Mux1/4  "[Qdotc, Qdotr]"
  Ts/1 -> Sum/2, Sum1/1  "Ts"
  Demux/2 -> Sum/1  "Tc"
  Mux/1 -> wallsurface/1
  Urad*emissivity/1 -> Mux/2, Sum2/2  "qdotr"
  Sum1/1 -> Urad*emissivity/1  "dTr"
  Demux/1 -> Terminator/1
  "[AIV]c"/1 -> Demux/1
  Demux/4 -> Terminator1/1
  Sum2/1 -> qdots/1
  Product1/1 -> Sum2/1, Mux/1  "qdotc"
  Sum/1 -> Product1/1, Abs/1, 1-D Lookup Table/1  "dTc"
  Demux/3 -> Sum1/2  "Tr"

== system carnot/Basic/Heat_Transfer/alfa_floor ==
  note: dynamic, convective heat transfer coefficients according to: Glück B.: Wärmeübergangskoeffizienten an thermisch aktiven Bauteiloberflächen
      | und der Übergang zu Basiskennlinien für die Wärmestromdichte; gi Gesundheits-Ingenieur; 128. Jahrgang 2007, Heft 1, Seiten 1-10
  note: (°C)
  note: (W/m^2)
  note: Convective and radiative heat transfer at the SURFACE OF A HORIZONTAL FLOOR
  note: s: surface
      | c: convective
      | r: radiative
  note: CONVENTION:
      | Qdot > 0 and qdots < 0, if Ts > T (heat flows from wall surface to room node),
      | Qdot < 0 and qdots > 0, if Ts < T (heat flows from room node to wall surface).
  Ts : Inport
  "[AIV]f" : Inport  Port=2
  Qdot sol : Inport  Port=3
  1-D Lookup Table : Lookup_n-D  NumberOfTableDimensions=1  BreakpointsForDimension1=[-10 -0.01 0.01 10]  BeginIndexSearchUsingPreviousIndexResult=on  Table=[0.54 0.54 2 2]  InternalRulePriority=Speed  RndMeth=Simplest  InputSameDT=on
  1/wallsurface : Gain  Gain=1/wallsurface  SaturateOnIntegerOverflow=on  OutDataTypeStr=Inherit: Same as input  ParamDataTypeStr=Inherit: Same as input
  Abs : Abs
  Constant : Constant  Value=0.31
  Demux : Demux  Outputs=[1 1 1 6]
  Ground : Ground
  Ground1 : Ground
  Ground2 : Ground
  Math Function : Math  Operator=pow  SaturateOnIntegerOverflow=on
  Mux : Mux  Inputs=[1 1]
  Mux1 : Mux  Inputs=[4 1 1 2 5]
  Product1 : Product  Inputs=3  SaturateOnIntegerOverflow=on  RndMeth=Zero  InputSameDT=on  OutDataTypeStr=Inherit: Same as first input
  Sum : Sum  Inputs=-+  SaturateOnIntegerOverflow=on  InputSameDT=on  OutDataTypeStr=Inherit: Same as first input
  Sum1 : Sum  Inputs=+-  SaturateOnIntegerOverflow=on  InputSameDT=on  OutDataTypeStr=Inherit: Same as first input
  Sum2 : Sum  Inputs=+--  SaturateOnIntegerOverflow=on  InputSameDT=on  OutDataTypeStr=Inherit: Same as first input
  Sum3 : Sum  Inputs=1  SaturateOnIntegerOverflow=on  InputSameDT=on  OutDataTypeStr=Inherit: Same as first input
  Terminator : Terminator
  Terminator1 : Terminator
  Urad*emissivity : Gain  Gain=5.6*emission_f  SaturateOnIntegerOverflow=on  OutDataTypeStr=Inherit: Same as input  ParamDataTypeStr=Inherit: Same as input
  active? : Gain  Gain=active  SaturateOnIntegerOverflow=on  OutDataTypeStr=Inherit: Same as input  ParamDataTypeStr=Inherit: Same as input
  wallsurface : Gain  Gain=wallsurface  SaturateOnIntegerOverflow=on  OutDataTypeStr=Inherit: Same as input  ParamDataTypeStr=Inherit: Same as input
  qdots : Outport
  "[S]f" : Outport  Port=2
  wires:
  Sum/1 -> Product1/1, 1-D Lookup Table/1, Abs/1  "dTc"
  Constant/1 -> Math Function/2
  Abs/1 -> Math Function/1
  1-D Lookup Table/1 -> Product1/2  "coeff_upwards_downwards"
  Math Function/1 -> Product1/3
  Demux/3 -> Sum1/2  "Tr"
  Product1/1 -> Mux/1, Sum2/2  "qdotc"
  Mux/1 -> wallsurface/1
  Urad*emissivity/1 -> Sum2/3, Mux/2  "qdotr"
  Sum1/1 -> Urad*emissivity/1  "dTr"
  Demux/1 -> Terminator/1
  "[AIV]f"/1 -> Demux/1
  Demux/4 -> Terminator1/1
  1/wallsurface/1 -> Sum2/1
  Ts/1 -> Sum1/1, Sum/2  "Ts"
  Sum2/1 -> qdots/1
  Demux/2 -> Sum/1  "Tc"
  wallsurface/1 -> Mux1/4, Sum3/1  "[Qdotc, Qdotr]"
  Qdot sol/1 -> 1/wallsurface/1
  Sum3/1 -> active?/1
  Ground/1 -> Mux1/1
  Ground1/1 -> Mux1/5
  Mux1/1 -> "[S]f"/1
  Ground2/1 -> Mux1/3
  active?/1 -> Mux1/2

== system carnot/Basic/Heat_Transfer/alfa_wall_in ==
  note: (°C)
  note: (W/m^2)
  note: Convective and radiative heat transfer at the INDOOR SURFACE of a VERTICAL OUTER WALL
  note: CONVENTION:
      | Qdot > 0 and qdots < 0, if Ts > T (heat flows from wall surface to room node),
      | Qdot < 0 and qdots > 0, if Ts < T (heat flows from room node to wall surface).
  note: s: surface
      | c: convective
      | r: radiative
  note: dynamic, convective heat transfer coefficients according to: Glück B.: Wärmeübergangskoeffizienten an thermisch aktiven Bauteiloberflächen
      | und der Übergang zu Basiskennlinien für die Wärmestromdichte; gi Gesundheits-Ingenieur; 128. Jahrgang 2007, Heft 1, Seiten 1-10
  Ts2 : Inport
  "[AIV]" : Inport  Port=2
  Abs : Abs
  Constant : Constant  Value=0.3
  Demux : Demux  Outputs=[1 1 1 6]
  Ground : Ground
  Ground1 : Ground
  Ground2 : Ground
  Math Function : Math  Operator=pow  SaturateOnIntegerOverflow=on
  Mux : Mux  Inputs=2
  Mux1 : Mux  Inputs=[4 1 1 2 5]
  Product1 : Product  SaturateOnIntegerOverflow=on  RndMeth=Zero  InputSameDT=on  OutDataTypeStr=Inherit: Same as first input
  Sum : Sum  Inputs=+-  SaturateOnIntegerOverflow=on  InputSameDT=on  OutDataTypeStr=Inherit: Same as first input
  Sum1 : Sum  Inputs=+-  SaturateOnIntegerOverflow=on  InputSameDT=on  OutDataTypeStr=Inherit: Same as first input
  Sum2 : Sum  Inputs=--  SaturateOnIntegerOverflow=on  InputSameDT=on  OutDataTypeStr=Inherit: Same as first input
  Sum3 : Sum  Inputs=1  SaturateOnIntegerOverflow=on  InputSameDT=on  OutDataTypeStr=Inherit: Same as first input
  Terminator : Terminator
  Terminator1 : Terminator
  Urad*emissivity : Gain  Gain=5.6*emission_in  SaturateOnIntegerOverflow=on  OutDataTypeStr=Inherit: Same as input  ParamDataTypeStr=Inherit: Same as input
  active layers : Gain  Gain=active  SaturateOnIntegerOverflow=on  OutDataTypeStr=Inherit: Same as input  ParamDataTypeStr=Inherit: Same as input
  gain : Gain  Gain=1.6  SaturateOnIntegerOverflow=on  OutDataTypeStr=Inherit: Same as input  ParamDataTypeStr=Inherit: Same as input
  wallsurface : Gain  Gain=wallsurface  SaturateOnIntegerOverflow=on  OutDataTypeStr=Inherit: Same as input  ParamDataTypeStr=Inherit: Same as input
  qdots2 : Outport
  "[S]" : Outport  Port=2
  wires:
  active layers/1 -> Mux1/2
  Ground2/1 -> Mux1/3
  Mux1/1 -> "[S]"/1
  Ground1/1 -> Mux1/5
  Ground/1 -> Mux1/1
  Sum3/1 -> active layers/1
  wallsurface/1 -> Sum3/1, Mux1/4  "[Qdotc, Qdotr]"
  Sum2/1 -> qdots2/1
  Demux/4 -> Terminator1/1
  "[AIV]"/1 -> Demux/1
  Demux/1 -> Terminator/1
  Demux/2 -> Sum/2  "Tc"
  Sum1/1 -> Urad*emissivity/1  "dTr"
  Urad*emissivity/1 -> Mux/2, Sum2/2  "qdotr"
  Mux/1 -> wallsurface/1
  Ts2/1 -> Sum/1, Sum1/1  "Ts"
  Demux/3 -> Sum1/2  "Tr"
  Product1/1 -> Sum2/1, Mux/1  "qdotc"
  Sum/1 -> Product1/1, Abs/1  "dTc"
  Constant/1 -> Math Function/2
  Abs/1 -> Math Function/1
  Math Function/1 -> gain/1
  gain/1 -> Product1/2

== system carnot/Basic/Heat_Transfer/alfa_wall_out ==
  note: dynamic, convective heat transfer coefficients according to: Glück B.: Wärmeübergangskoeffizienten an thermisch aktiven Bauteiloberflächen
      | und der Übergang zu Basiskennlinien für die Wärmestromdichte; gi Gesundheits-Ingenieur; 128. Jahrgang 2007, Heft 1, Seiten 1-10
  note: Convective heat transfer outer surface according to EN 6946
      | Radiative heat transfer to the ground is limited by a view of 0.25, i.e. view factor to the sky is 0.75 (Frohner, 2005)
  note: Convective and radiative heat transfer at the WEATHER EXPOSED SURFACE OF AN OUTER WALL
  note: s: surface
      | c: convective
      | r: radiative
      | h: in height
      | t: tilted surface
  note: CONVENTION:
      | qdots < 0, if Ts > T, heat flows from window surface (resp. room node) to ambient,
      | qdots > 0, if Ts < T, heat flows from ambient to window surface (resp. room node).
  note: wind dependent heat transfer EN 6946
  note: (3 = Sky model Perez)
  WDB : Inport
  Ts1 : Inport  Port=2
  Bias : Bias  Bias=4
  Bus Selector : BusSelector  OutputSignals=Wind_Speed,Temperature_Ambient,Temperature_Sky_Radiation
  Bus Selector1 : BusSelector  OutputSignals=Solar_Radiation_direct_surface,Solar_Radiation_diffuse_surface  OutputAsBus=on
  Gain : Gain  Gain=4
  Product2 : Product  SaturateOnIntegerOverflow=on  RndMeth=Zero  InputSameDT=on  OutDataTypeStr=Inherit: Same as first input
  Radiation_on_Inclined_Surface : $bdroot/Weather/Radiation_on_Inclined_Surface  sky=Perez 1990  reflect=0.2
  Sum : Sum  Inputs=+-  SaturateOnIntegerOverflow=on  InputSameDT=on  OutDataTypeStr=Inherit: Same as first input
  Sum1 : Sum  Inputs=1  SaturateOnIntegerOverflow=on  InputSameDT=on  OutDataTypeStr=Inherit: Same as first input
  Sum2 : Sum  Inputs=+++  SaturateOnIntegerOverflow=on  InputSameDT=on  OutDataTypeStr=Inherit: Same as first input
  absorption_out : Gain  Gain=absorption_out  SaturateOnIntegerOverflow=on  OutDataTypeStr=Inherit: Same as input  ParamDataTypeStr=Inherit: Same as input
  position : Constant  Value=pos
  wall_out_ IR_radiation : $bdroot/Basic/Heat_Transfer/wall_out_IR_radiation  SystemSampleTime=-1
  qdots1 : Outport
  wires:
  Gain/1 -> Bias/1
  Bus Selector/1 -> Gain/1  "<Wind_Speed>"
  Bus Selector/3 -> wall_out_ IR_radiation/2  "<Temperature_Sky_Radiation>"
  Bus Selector/2 -> wall_out_ IR_radiation/1, Sum/1  "<Temperature_Ambient>"
  Sum/1 -> Product2/1  "dTc"
  WDB/1 -> Radiation_on_Inclined_Surface/1, Bus Selector/1
  Sum2/1 -> qdots1/1
  Ts1/1 -> wall_out_ IR_radiation/3, Sum/2  "Ts (outer wall surface)"
  Sum1/1 -> absorption_out/1
  Bias/1 -> Product2/2  "alfa"
  absorption_out/1 -> Sum2/3  "qdot,sun"
  Product2/1 -> Sum2/1  "qdot_conv"
  wall_out_ IR_radiation/1 -> Sum2/2  "qdot_rad"
  Bus Selector1/1 -> Sum1/1
  Radiation_on_Inclined_Surface/1 -> Bus Selector1/1
  position/1 -> Radiation_on_Inclined_Surface/2

== system carnot/Basic/Heat_Transfer/alfa_window_in ==
  note: (W/m^2)
  note: CONVENTION:
      | Qdot > 0 and qdots < 0, if Ts > T (heat flows from wall surface to room node),
      | Qdot < 0 and qdots > 0, if Ts < T (heat flows from room node to wall surface).
  note: s: surface
      | c: convective
      | r: radiative
  note: WINDOW = FRAME + GLASS
  note: Convective and radiative heat transfer at the INDOOR SURFACE OF A VERTICAL WINDOW
      | with 1-4 layers (each 3 ... 8 mm thick)
  note: (°C)
  Ts2 : Inport
  "[sun_t]" : Inport  Port=2
  "[AIV]" : Inport  Port=3
  WDB : Inport  Port=4
  control : Inport  Port=5
  " glass surface" : Gain  Gain=(1-frame)*wallsurface  SaturateOnIntegerOverflow=on  OutDataTypeStr=Inherit: Same as input  ParamDataTypeStr=Inherit: Same as input
  Demux : Demux  Outputs=[1 1 1 6]
  Gain : Gain  Gain=1-frame
  Ground : Ground
  Ground1 : Ground
  Mux : Mux  Inputs=2
  Mux1 : Mux  Inputs=[1 5 2 5]
  Shading : Subsystem
  Subsystem : Subsystem
  Sum : Sum  Inputs=-+  SaturateOnIntegerOverflow=on  InputSameDT=on  OutDataTypeStr=Inherit: Same as first input
  Sum1 : Sum  Inputs=+-  SaturateOnIntegerOverflow=on  InputSameDT=on  OutDataTypeStr=Inherit: Same as first input
  Sum2 : Sum  Inputs=--+  SaturateOnIntegerOverflow=on  InputSameDT=on  OutDataTypeStr=Inherit: Same as first input
  Terminator : Terminator
  Terminator1 : Terminator
  Urad*emissivity : Gain  Gain=5.6*emission_in  SaturateOnIntegerOverflow=on  OutDataTypeStr=Inherit: Same as input  ParamDataTypeStr=Inherit: Same as input
  u_convection : Gain  Gain=2.5  SaturateOnIntegerOverflow=on  OutDataTypeStr=Inherit: Same as input  ParamDataTypeStr=Inherit: Same as input
  window surface : Gain  Gain=wallsurface  SaturateOnIntegerOverflow=on  OutDataTypeStr=Inherit: Same as input  ParamDataTypeStr=Inherit: Same as input
  qdots2 : Outport
  "[S]" : Outport  Port=2
  wires:
  Subsystem/2(qdot_sol) -> " glass surface"/1
  Subsystem/1(qdot_abs) -> Gain/1
  Shading/4(f_tau) -> Subsystem/5(In5)
  Shading/3(f_g) -> Subsystem/4(In4)
  Shading/2(f_dfu) -> Subsystem/3(In3)
  Shading/1(f_dir) -> Subsystem/2(In2)
  "[sun_t]"/1 -> Subsystem/1(sun_t)
  WDB/1 -> Shading/1(WDB)
  control/1 -> Shading/2(control)
  Ground1/1 -> Mux1/4
  Ground/1 -> Mux1/2
  Mux1/1 -> "[S]"/1
  Sum2/1 -> qdots2/1
  Demux/4 -> Terminator1/1
  "[AIV]"/1 -> Demux/1
  Demux/1 -> Terminator/1
  Mux/1 -> window surface/1
  Sum1/1 -> Urad*emissivity/1  "dTr"
  Ts2/1 -> Sum/2, Sum1/1  "Ts"
  Urad*emissivity/1 -> Sum2/2, Mux/2  "qdotr"
  u_convection/1 -> Mux/1, Sum2/1  "qdotc"
  " glass surface"/1 -> Mux1/1  "Qdot_sol"
  window surface/1 -> Mux1/3  "[Qdotc, Qdotr]"
  Demux/2 -> Sum/1  "Tc"
  Sum/1 -> u_convection/1  "dTc"
  Demux/3 -> Sum1/2  "Tr"
  Gain/1 -> Sum2/3

== system carnot/Basic/Heat_Transfer/alfa_window_out ==
  note: CONVENTION:
      | qdots < 0, if Ts > T, heat flows from window surface (resp. room node) to ambition,
      | qdots > 0, if Ts < T, heat flows from ambition to window surface (resp. room node).
  note: s: surface
      | c: convective
      | r: radiative
      | h: in height
      | t: tilted surface
  note: Convective and radiative heat transfer at the OUTDOOR SURFACE OF A VERTICAL WINDOW
  note: WINDOW = FRAME + GLASS
  WDB : Inport
  g : Inport  Port=2
  Ts1 : Inport  Port=3
  Bias : Bias  Bias=2.8
  Bus Selector : BusSelector  OutputSignals=Wind_Speed,Temperature_Ambient,Temperature_Sky_Radiation
  Bus Selector1 : BusSelector  OutputSignals=Incidence_Angle_sun,Solar_Radiation_direct_surface,Solar_Radiation_diffuse_surface
  Gain : Gain  Gain=3
  Mux1 : Mux  Inputs=2
  Mux2 : Mux  Inputs=2
  Product6 : Product  SaturateOnIntegerOverflow=on  InputSameDT=on  OutDataTypeStr=Inherit: Same as first input
  Product7 : Product  SaturateOnIntegerOverflow=on  InputSameDT=on  OutDataTypeStr=Inherit: Same as first input
  Radiation_on_Inclined_Surface : $bdroot/Weather/Radiation_on_Inclined_Surface  sky=Perez 1990  reflect=0.2
  Sum : Sum  Inputs=+-  SaturateOnIntegerOverflow=on  InputSameDT=on  OutDataTypeStr=Inherit: Same as first input
  Sum2 : Sum  Inputs=+++  SaturateOnIntegerOverflow=on  InputSameDT=on  OutDataTypeStr=Inherit: Same as first input
  Sum3 : Sum  SaturateOnIntegerOverflow=on  InputSameDT=on  OutDataTypeStr=Inherit: Same as first input
  absorption_out * frame : Gain  Gain=absorption_out * frame  SaturateOnIntegerOverflow=on  OutDataTypeStr=Inherit: Same as input  ParamDataTypeStr=Inherit: Same as input
  position : Constant  Value=pos
  wall_out_ IR_radiation : $bdroot/Basic/Heat_Transfer/wall_out_IR_radiation  SystemSampleTime=-1
  "[sun_t]" : Outport
  qdots1 : Outport  Port=2
  wires:
  Gain/1 -> Bias/1
  Bus Selector/1 -> Gain/1  "<Wind_Speed>"
  Bus Selector/3 -> wall_out_ IR_radiation/2  "<Temperature_Sky_Radiation>"
  Bus Selector/2 -> Sum/1, wall_out_ IR_radiation/1  "<Temperature_Ambient>"
  Bus Selector1/3 -> Sum3/2, Mux2/2  "<Solar_Radiation_diffuse_surface>"
  Mux2/1 -> Product6/1
  Product6/1 -> Mux1/2
  Sum/1 -> Product7/1  "dTc"
  WDB/1 -> Bus Selector/1, Radiation_on_Inclined_Surface/1
  Bus Selector1/1 -> Mux1/1  "<Incidence_Angle_sun>"
  Sum3/1 -> absorption_out * frame/1
  Sum2/1 -> qdots1/1
  g/1 -> Product6/2
  absorption_out * frame/1 -> Sum2/3
  Bus Selector1/2 -> Sum3/1, Mux2/1  "<Solar_Radiation_direct_surface>"
  Mux1/1 -> "[sun_t]"/1
  Ts1/1 -> wall_out_ IR_radiation/3, Sum/2  "Ts (outer wall surface)"
  wall_out_ IR_radiation/1 -> Sum2/2  "qdotr"
  Bias/1 -> Product7/2  "alfa"
  Product7/1 -> Sum2/1  "qdot,conv"
  position/1 -> Radiation_on_Inclined_Surface/2
  Radiation_on_Inclined_Surface/1 -> Bus Selector1/1

== system carnot/Basic/Heat_Transfer/wall_out_IR_radiation ==
  note: Wall has a view on 50% ground and 50% sky (true for vertical walls).
      | Longwave radiation emissiviy of ground and sky assumed to be 1.
  Tamb : Inport
  Tsky : Inport  Port=2
  Twall : Inport  Port=3
  Bias : Bias  Bias=273.15
  Gain : Gain  Gain=[-1 0.5 0.5]*emission_out*5.67e-8
  Math Function : Math  Operator=square  SaturateOnIntegerOverflow=on
  Math Function1 : Math  Operator=square  SaturateOnIntegerOverflow=on
  Mux : Mux  Inputs=3
  Sum : Sum  Inputs=1  SaturateOnIntegerOverflow=on  InputSameDT=on  OutDataTypeStr=Inherit: Same as first input
  qrad : Outport
  wires:
  Tsky/1 -> Mux/2
  Tamb/1 -> Mux/3
  Sum/1 -> qrad/1
  Twall/1 -> Mux/1
  Bias/1 -> Math Function/1
  Mux/1 -> Bias/1
  Math Function/1 -> Math Function1/1
  Gain/1 -> Sum/1
  Math Function1/1 -> Gain/1

== system carnot/Basic/Hydraulics/ElectricConsumptionPump ==
  mdot : Inport
  Ctrl : Inport  Port=2
  Add : Sum  Inputs=3
  Compare To Zero : simulink/Logic and Bit Operations/Compare To Zero  relop=>  OutDataTypeStr=boolean
  Constant : Constant  Value=e0
  Linear : Gain  Gain=e1
  Math Function : Math  Operator=square  SaturateOnIntegerOverflow=on
  Product : Product
  Quadratic : Gain  Gain=e2
  Pel : Outport
  wires:
  Compare To Zero/1 -> Product/2
  Add/1 -> Product/1  "Pel"
  Ctrl/1 -> Compare To Zero/1
  Constant/1 -> Add/3
  Product/1 -> Pel/1  "Pel"
  Math Function/1 -> Quadratic/1
  Linear/1 -> Add/2
  mdot/1 -> Math Function/1, Linear/1
  Quadratic/1 -> Add/1

== system carnot/Basic/Hydraulics/Flow_Mixer_basic ==
  THB1 : Inport
  THB2 : Inport  Port=2
  clq : Inport  Port=3
  Bus Assignment : BusAssignment  AssignedSignals=ID,Temperature,MassFlow,Pressure,FluidType,FluidMix,DiameterLastPiece,DPConstant,DPLinear,DPQuadratic
  Bus Selector : BusSelector  OutputSignals=ID
  Bus Selector2 : BusSelector  OutputSignals=Pressure  OutputAsBus=on
  Bus Selector3 : BusSelector  OutputSignals=FluidType  OutputAsBus=on
  Bus Selector4 : BusSelector  OutputSignals=DiameterLastPiece  OutputAsBus=on
  Bus Selector6 : BusSelector  OutputSignals=ID
  Bus Selector8 : BusSelector  OutputSignals=Pressure  OutputAsBus=on
  Bus Selector9 : BusSelector  OutputSignals=DiameterLastPiece  OutputAsBus=on
  Demux1 : Demux  Outputs=3
  MinMax : MinMax  Function=max  Inputs=2
  MinMax1 : MinMax  Inputs=2
  Mix_T_Mdot : $bdroot/Basic/Hydraulics/Mix_T_Mdot  mixcalc=Tmix = (mdot1*T1 + mdot2*T2)/(mdot1+mdot2)
  S-Function : S-Function  FunctionName=mix_flow  SFunctionDeploymentMode=off  EnableBusSupport=off
  Subsystem : Subsystem
  Subsystem1 : Subsystem
  Subsystem2 : Subsystem
  average_1 : Subsystem
  decrease_ID1 : Subsystem
  decrease_ID2 : Subsystem
  THB : Outport
  ID1 : Outport  Port=2
  ID2 : Outport  Port=3
  fdiv : Outport  Port=4
  wires:
  Subsystem1/1(IDclq) -> S-Function/1
  Subsystem/1(clq) -> S-Function/3
  S-Function/2 -> fdiv/1
  clq/1 -> Subsystem/1(clq_bus)
  Bus Assignment/1 -> THB/1
  Subsystem2/1(IDclq) -> S-Function/2
  Bus Selector2/1 -> MinMax1/1  "p"
  Mix_T_Mdot/2 -> Bus Assignment/4
  Mix_T_Mdot/3 -> Bus Assignment/7
  Mix_T_Mdot/1 -> Bus Assignment/3  "T"
  S-Function/1 -> Demux1/1
  Demux1/3 -> Bus Assignment/11  "qua"
  Demux1/2 -> Bus Assignment/10  "lin"
  Demux1/1 -> Bus Assignment/9  "con"
  MinMax1/1 -> Bus Assignment/5  "p"
  average_1/1(Out1) -> Bus Assignment/8
  Bus Selector9/1 -> average_1/2(In2)  "diameter"
  Bus Selector4/1 -> average_1/1(In1)  "diameter"
  Bus Selector8/1 -> MinMax1/2  "p"
  Bus Selector6/1 -> ID2/1, decrease_ID2/1(In1)  "<ID>"
  THB2/1 -> Bus Selector6/1, Subsystem2/1(THB), Bus Selector8/1, Bus Selector9/1, Mix_T_Mdot/2
  Bus Selector3/1 -> Bus Assignment/6  "fluid"
  MinMax/1 -> Bus Assignment/2  "ID"
  decrease_ID2/1(Out1) -> MinMax/2
  decrease_ID1/1(Out1) -> MinMax/1
  Bus Selector/1 -> decrease_ID1/1(In1), ID1/1  "<ID>"
  THB1/1 -> Bus Selector4/1, Subsystem1/1(THB), Mix_T_Mdot/1, Bus Selector3/1, Bus Selector2/1, Bus Selector/1, Bus Assignment/1
